simulink model "etc_system"  (R2024a)
settings: Solver=VariableStepAuto  StartTime=0.0  StopTime=10.0  RelTol=1e-3
PreLoadFcn:
  | % Load controller parameters
  | etc_PI_data
  | 
  | % Load throttle parameters
  | etc_plant_data
undefined symbols (not defined in the file or in its folder): J, Kd, Ki, Km, Kp, Ks, theta_eq, Ts
libraries: SignalEditorBlockLib x1
settings Model: Creator=bneiswan  LastModifiedBy=bneiswan
settings RTWCC: GPUComputeCapability=3.5

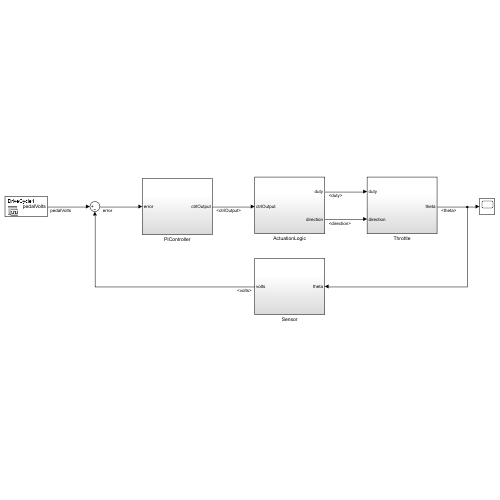
[thumbnail: Simulink's stored preview of the top-level diagram]
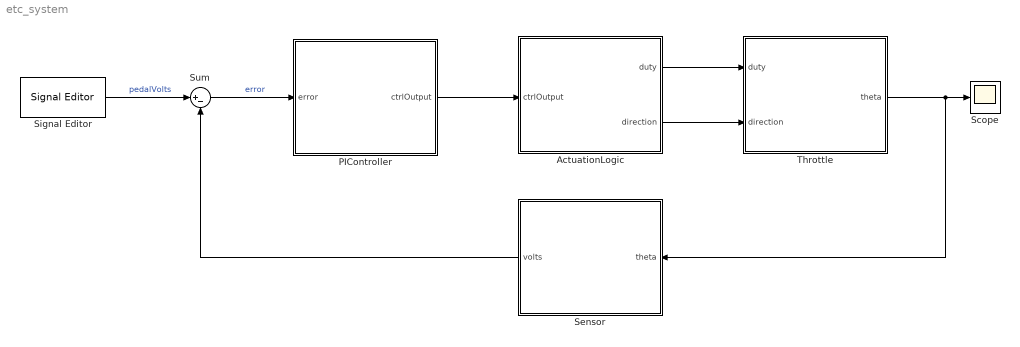
== system etc_system ==
  ActuationLogic : Subsystem
  PIController : Subsystem
  Scope : Scope
  Sensor : Subsystem
  Signal Editor : SignalEditorBlockLib/Signal Editor  FileName=driveCycleData.mat  ActiveScenario=DriveCycle1  ActiveSignal=pedalVolts  IsBus=off  OutputBusObjectStr=Bus: BusObject  SampleTime=0  Interpolate=off  ZeroCross=off  OutputAfterFinalValue=Setting to zero  Unit=inherit  PreserveSignalName=on  ApplySigPropsToAllScenarios=on  ApplySigPropsToAllSignals=off
  Sum : Sum  Inputs=|+-
  Throttle : Subsystem
  wires:
  Sensor/1(volts) -> Sum/2
  Signal Editor/1 -> Sum/1  "pedalVolts"
  Sum/1 -> PIController/1(error)  "error"
  ActuationLogic/1(duty) -> Throttle/1(duty)
  ActuationLogic/2(direction) -> Throttle/2(direction)
  PIController/1(ctrlOutput) -> ActuationLogic/1(ctrlOutput)
  Throttle/1(theta) -> Sensor/1(theta), Scope/1

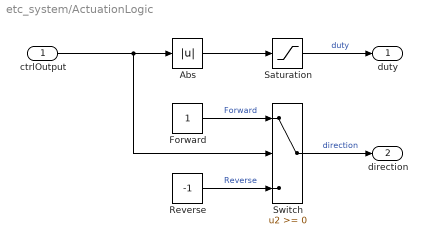
== system etc_system/ActuationLogic ==
  ctrlOutput : Inport
  Abs : Abs  SaturateOnIntegerOverflow=off
  Forward : Constant  OutDataTypeStr=double
  Reverse : Constant  Value=-1  OutDataTypeStr=double
  Saturation : Saturate  UpperLimit=1  LowerLimit=0
      settings: AttributesFormatString=%<LowerLimit> < duty < %<UpperLimit>
  Switch : Switch  SaturateOnIntegerOverflow=off  InputSameDT=off
      settings: AttributesFormatString=Criteria: %<Criteria>\nThreshold: %<Threshold>
  duty : Outport  VectorParamsAs1DForOutWhenUnconnected=off
  direction : Outport  Port=2  VectorParamsAs1DForOutWhenUnconnected=off
  wires:
  Saturation/1 -> duty/1  "duty"
  Forward/1 -> Switch/1  "Forward"
  Reverse/1 -> Switch/3  "Reverse"
  Abs/1 -> Saturation/1
  Switch/1 -> direction/1  "direction"
  ctrlOutput/1 -> Switch/2, Abs/1

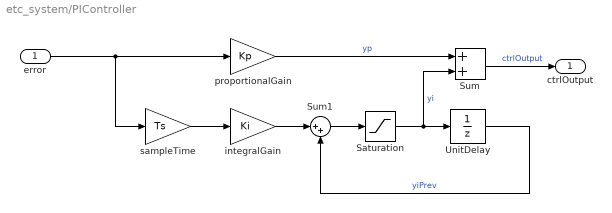
== system etc_system/PIController ==
  error : Inport
  Saturation : Saturate  UpperLimit=1  LowerLimit=-1
      settings: AttributesFormatString=Max: %<UpperLimit>\nMin: %<LowerLimit>
  Sum : Sum  InputSameDT=on  SaturateOnIntegerOverflow=on  OutDataTypeStr=Inherit: Same as first input
  Sum1 : Sum  Inputs=|++  InputSameDT=on  SaturateOnIntegerOverflow=on  OutDataTypeStr=Inherit: Same as first input
  UnitDelay : UnitDelay  SampleTime=Ts  HasFrameUpgradeWarning=on
      settings: AttributesFormatString=yi0 = %<X0>\nSample time = %<SampleTime>
  integralGain : Gain  Gain=Ki  SaturateOnIntegerOverflow=on  OutDataTypeStr=Inherit: Same as input  ParamDataTypeStr=Inherit: Same as input
  proportionalGain : Gain  Gain=Kp  SaturateOnIntegerOverflow=on  OutDataTypeStr=Inherit: Same as input  ParamDataTypeStr=Inherit: Same as input
  sampleTime : Gain  Gain=Ts  SaturateOnIntegerOverflow=on  OutDataTypeStr=Inherit: Same as input  ParamDataTypeStr=Inherit: Same as input
  ctrlOutput : Outport  VectorParamsAs1DForOutWhenUnconnected=off
  wires:
  sampleTime/1 -> integralGain/1
  error/1 -> proportionalGain/1, sampleTime/1
  integralGain/1 -> Sum1/1
  Saturation/1 -> Sum/2, UnitDelay/1  "yi"
  UnitDelay/1 -> Sum1/2  "yiPrev"
  Sum/1 -> ctrlOutput/1  "ctrlOutput"
  proportionalGain/1 -> Sum/1  "yp"
  Sum1/1 -> Saturation/1

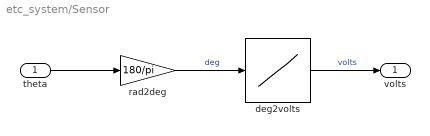
== system etc_system/Sensor ==
  theta : Inport
  deg2volts : Lookup_n-D  NumberOfTableDimensions=1  BreakpointsForDimension1=[0 90]  Table=[0.5 4.5]  RndMeth=Simplest
  rad2deg : Gain  Gain=180/pi
  volts : Outport  VectorParamsAs1DForOutWhenUnconnected=off
  wires:
  rad2deg/1 -> deg2volts/1  "deg"
  deg2volts/1 -> volts/1  "volts"
  theta/1 -> rad2deg/1

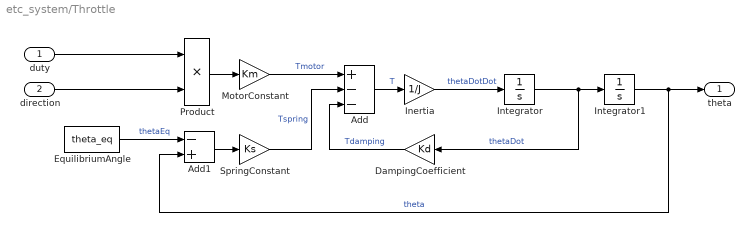
== system etc_system/Throttle ==
  duty : Inport
  direction : Inport  Port=2
  Add : Sum  Inputs=+--
  Add1 : Sum  Inputs=-+
  DampingCoefficient : Gain  Gain=Kd
  EquilibriumAngle : Constant  Value=theta_eq
  Inertia : Gain  Gain=1/J
  Integrator : Integrator
      settings: AttributesFormatString=I.C. = %<InitialCondition>
  Integrator1 : Integrator  InitialCondition=theta_eq  LimitOutput=on  UpperSaturationLimit=pi/2  LowerSaturationLimit=0
      settings: AttributesFormatString=|
      | I.C. = %<InitialCondition>
      | %<LowerSaturationLimit><=theta<=%<UpperSaturationLimit>
  MotorConstant : Gain  Gain=Km
  Product : Product
  SpringConstant : Gain  Gain=Ks
  theta : Outport
  wires:
  DampingCoefficient/1 -> Add/3  "Tdamping"
  SpringConstant/1 -> Add/2  "Tspring"
  EquilibriumAngle/1 -> Add1/1  "thetaEq"
  Integrator/1 -> Integrator1/1, DampingCoefficient/1  "thetaDot"
  Integrator1/1 -> theta/1, Add1/2  "theta"
  Inertia/1 -> Integrator/1  "thetaDotDot"
  Product/1 -> MotorConstant/1
  Add1/1 -> SpringConstant/1
  Add/1 -> Inertia/1  "T"
  MotorConstant/1 -> Add/1  "Tmotor"
  duty/1 -> Product/1
  direction/1 -> Product/2
